simulink model "ex_househeat_modeling"  (R2023b)
settings: Solver=VariableStepAuto  StartTime=0.0  StopTime=24  FixedStep=1  RelTol=1e-3  EnableMultiTasking=on
settings Model: Creator=The MathWorks, Inc.  LastModifiedBy=The MathWorks, Inc.
settings SolverCC: AlgebraicLoopSolver=TrustRegion  MinimalZcImpactIntegration=on
settings DataIOCC: LimitDataPoints=on  SaveFormat=Array  ReturnWorkspaceOutputs=off
settings OptimizationCC: ReuseModelBlockBuffer=off  LifeSpan=inf
settings DebuggingCC: UnconnectedInputMsg=warning  UnconnectedOutputMsg=warning  UnconnectedLineMsg=warning  SFUnexpectedBacktrackingDiag=warning  SFNoUnconditionalDefaultTransitionDiag=warning  SFExecutionAtInitializationDiag=none  ArithmeticOperatorsInVariantConditions=warning
settings HardwareCC: ProdBitPerPointer=32  ProdBitPerSizeT=32  ProdBitPerPtrDiffT=32  ProdLargestAtomicFloat=None  ProdIntDivRoundTo=Undefined  ProdEndianess=Unspecified  ProdWordSize=32  ProdHWDeviceType=32-bit Generic
settings ModelReferenceCC: EnableRefExpFcnMdlSchedulingChecks=on  PropagateSignalLabelsOutOfModel=off
settings SFSimCC: SimUseLocalCustomCode=off  CustomCodeUndefinedFunction=UseInterfaceOnly
settings RTWCC: RTWUseLocalCustomCode=off
settings CodeAppCC: StateflowObjectComments=on
settings GRTTargetCC: TargetLangStandard=C89/C90 (ANSI)
settings ConfigComp: CovMetricSettings=dw  CovSaveCumulativeToWorkspaceVar=on  CovSaveSingleToWorkspaceVar=on  CovExternalEMLEnable=off  CovSFcnEnable=off

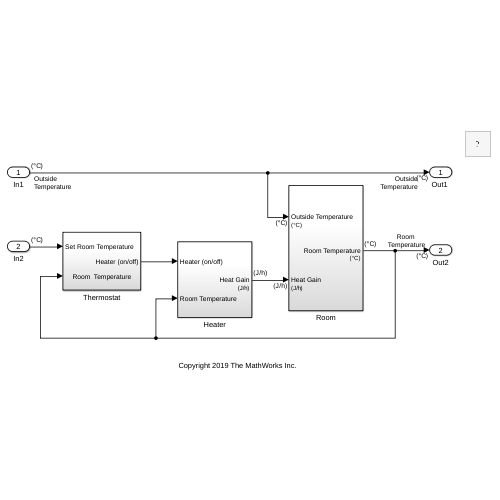
[thumbnail: Simulink's stored preview of the top-level diagram]
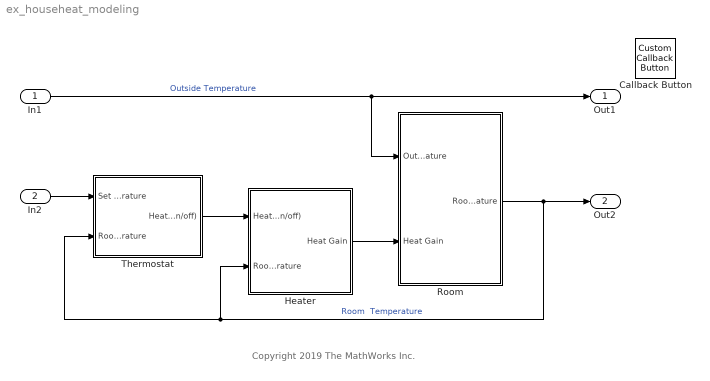
== system ex_househeat_modeling ==
  note: Copyright 2019 The MathWorks Inc.
  In1 : Inport  Unit=°C
  In2 : Inport  Port=2  Unit=°C
  Callback Button : CustomCallbackButton  Configuration="{\"components\":[{\"name\":\"BackgroundImageComponent\",\"settings\":{\"image\":{\"size\":[0,0],\"src\":\"default\",\"srcOrientation\":\"Right\"},\"position\":[0,0,1,1]}},{\"name\":\"ButtonStateComponent\",\"settings\":{\"buttonType\":\"momentary\",\"clickFcn\":\"showExample('simulink\\/OpenCompletedHouseSystemModelExample')\",\"onValue\":1,\"position\":[0,0,1,1],\"pressDelay\":\"500\",\"pressFcn\":\"\",\"repeatInterval\":\"0\",\"states\":[{\"horizontalAlignment\":\"center\",\"image\":{\"position\":[0,0,1,1],\"size\":[1,1],\"src\":\"default\",\"srcOrientation\":\"Right\"},\"label\":{\"color\":[0.01176470588,0.01176470588,0.01176470588,1],\"icon\":{\"size\":[0,0],\"src\":\"default\",\"srcOrientation\":\"Right\"},\"iconPlacement\":\"left\",\"opacity\":1,\"show\":true,\"text\":{\"content\":\"?\",\"font\":\"Helvetica\",\"fontSize\":14.735309999999998}},\"labelOffset\":[0,0],\"verticalAlignment\":\"middle\"},{\"horizontalAlignment\":\"center\",\"image\":{\"position\":[0,0,1,1],\"size\":[1,1],\"src\":\"default\",\"srcOrientation\":\"Right\"},\"label\":{\"color\":[0.01176470588,0.01176470588,0.01176470588,1],\"icon\":{\"size\":[0,0],\"src\":\"default\",\"srcOrientation\":\"Right\"},\"iconPlacement\":\"left\",\"opacity\":1,\"show\":true,\"text\":{\"content\":\"?\",\"font\":\"Helvetica\",\"fontSize\":14.735309999999998}},\"labelOffset\":[0,0],\"verticalAlignment\":\"middle\"},{\"horizontalAlignment\":\"center\",\"image\":{\"position\":[0,0,1,1],\"size\":[1,1],\"src\":\"default\",\"srcOrientation\":\"Right\"},\"label\":{\"color\":[0.01176470588,0.01176470588,0.01176470588,1],\"icon\":{\"size\":[0,0],\"src\":\"default\",\"srcOrientation\":\"Right\"},\"iconPlacement\":\"left\",\"opacity\":1,\"show\":true,\"text\":{\"content\":\"?\",\"font\":\"Helvetica\",\"fontSize\":14.735309999999998}},\"labelOffset\":[0,0],\"verticalAlignment\":\"middle\"},{\"horizontalAlignment\":\"center\",\"image\":{\"position\":[0,0,1,1],\"size\":[1,1],\"src\":\"default\",\"srcOrientation\":\"Right\"},\"label\":{\"color\":[0.01176470588,0.01176470588,0.01176470588,1],\"icon\":{\"size\":[0,0],\"src\":\"default\",\"srcOrientation\":\"Right\"},\"iconPlacement\":\"left\",\"opacity\":1,\"show\":true,\"text\":{\"content\":\"?\",\"font\":\"Helvetica\",\"fontSize\":14.735309999999998}},\"labelOffset\":[0,0],\"verticalAlignment\":\"middle\"}]}},{\"name\":\"ForegroundImageComponent\",\"settings\":{\"image\":{\"size\":[0,0],\"src\":\"default\",\"srcOrientation\":\"Right\"},\"isForeground\":1,\"position\":[0,0,1,1]}}],\"settings\":{\"BindingType\":\"standalone\",\"backgroundColor\":[244,244,244,1],\"backgroundOffset\":0,\"backgroundOpacity\":1,\"fixedAspectRatio\":\"off\",\"foregroundColor\":[0.01176470588,0.01176470588,0.01176470588,1],\"migratedFromLegacy\":true,\"useBackgroundColor\":true,\"variant\":\"callback\",\"version\":\"R2023a\"},\"type\":\"Button\"}"  CustomBackgroundColor="{\"color\":[0.9568627451,0.9568627451,0.9568627451],\"show\":true}"
  Heater : Subsystem
  Room : Subsystem
  Thermostat : Subsystem
  "Out1 " : Outport  Unit=°C  VectorParamsAs1DForOutWhenUnconnected=off
  Out2 : Outport  Port=2  Unit=°C  VectorParamsAs1DForOutWhenUnconnected=off
  wires:
  Thermostat/1(Heater (on/off)) -> Heater/1(Heater (on/off))
  Heater/1(Heat Gain) -> Room/2("Heat Gain ")
  Room/1(Room Temperature) -> Out2/1, Heater/2(Room Temperature), Thermostat/2("    Room Temperature")  "Room  Temperature"
  In2/1 -> Thermostat/1(Set Room Temperature)
  In1/1 -> Room/1(Outside Temperature), "Out1 "/1  "Outside Temperature"

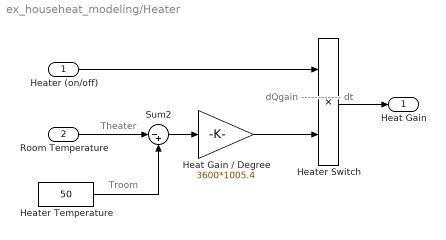
== system ex_househeat_modeling/Heater ==
  note: dQgain
      | ------------
      |    dt
  note: Troom
  note: Theater
  Heater (on/off) : Inport
  Room Temperature : Inport  Port=2
  Heat Gain / Degree : Gain  Gain=3600*1005.4
  Heater Switch : Product  RndMeth=Zero
  Heater Temperature : Constant  Value=50
  Sum2 : Sum  Inputs=|-+
  Heat Gain : Outport  Unit=joule/hour  VectorParamsAs1DForOutWhenUnconnected=off
  wires:
  Heater Temperature/1 -> Sum2/2
  Room Temperature/1 -> Sum2/1
  Sum2/1 -> Heat Gain / Degree/1
  Heat Gain / Degree/1 -> Heater Switch/2
  Heater (on/off)/1 -> Heater Switch/1
  Heater Switch/1 -> Heat Gain/1

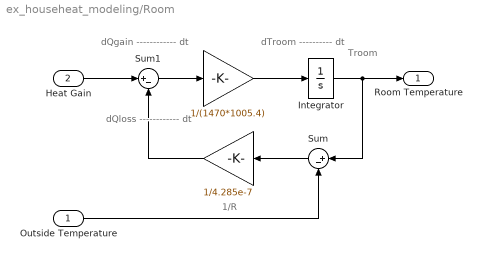
== system ex_househeat_modeling/Room ==
  note: 1/R
  note: Troom
  note: dQloss
      | ------------
      |      dt
  note: dQgain
      | ------------
      |      dt
  note: dTroom
      | ----------
      |     dt
  Outside Temperature : Inport  Unit=°C
  "Heat Gain " : Inport  Port=2  Unit=joule/h
  " " : Gain  Gain=1/4.285e-7  SaturateOnIntegerOverflow=on  OutDataTypeStr=Inherit: Same as input  ParamDataTypeStr=Inherit: Same as input
  "  " : Gain  Gain=1/(1470*1005.4)  SaturateOnIntegerOverflow=on  OutDataTypeStr=Inherit: Same as input  ParamDataTypeStr=Inherit: Same as input
  Integrator : Integrator  InitialCondition=20
  Sum : Sum  Inputs=|+-
  Sum1 : Sum  Inputs=|+-  InputSameDT=on  SaturateOnIntegerOverflow=on  OutDataTypeStr=Inherit: Same as first input
  Room Temperature : Outport  Unit=°C  VectorParamsAs1DForOutWhenUnconnected=off
  wires:
  "Heat Gain "/1 -> Sum1/1
  Sum1/1 -> "  "/1
  "  "/1 -> Integrator/1
  Integrator/1 -> Sum/1, Room Temperature/1
  " "/1 -> Sum1/2
  Sum/1 -> " "/1
  Outside Temperature/1 -> Sum/2

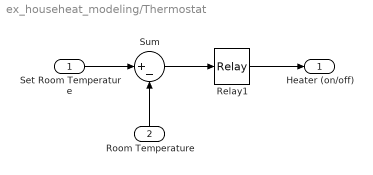
== system ex_househeat_modeling/Thermostat ==
  Set Room Temperature : Inport
  "    Room Temperature" : Inport  Port=2
  Relay1 : Relay  OnSwitchValue=2  OffSwitchValue=-2
  Sum : Sum  Inputs=|+-  InputSameDT=on  SaturateOnIntegerOverflow=on  OutDataTypeStr=Inherit: Same as first input
  Heater (on/off) : Outport  VectorParamsAs1DForOutWhenUnconnected=off
  wires:
  Set Room Temperature/1 -> Sum/1
  Relay1/1 -> Heater (on/off)/1
  Sum/1 -> Relay1/1
  "    Room Temperature"/1 -> Sum/2
